simulink model "simulink_model"  (R2019a)
settings: Solver=VariableStepAuto  StartTime=0.0  StopTime=30  RelTol=1e-3
values from neighbouring files (symbols this model uses):
  Kd = 0.28409    [step_10_and_onward.m]
  Ki = 0.05    [step_10_and_onward.m]
  Kp = 1    [P_design.m]    (also in step_10_and_onward.m = 3.12954)
libraries: simulink x1
settings Model: Creator=zma70  LastModifiedBy=zma70

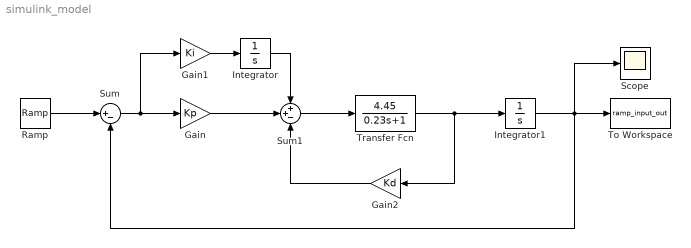
== system simulink_model ==
  Gain : Gain  Gain=Kp
  Gain1 : Gain  Gain=Ki
  Gain2 : Gain  Gain=Kd
  Integrator : Integrator
  Integrator1 : Integrator
  Ramp : simulink/Sources/Ramp  slope=1  start=0  InitialOutput=0
  Scope : Scope
  Sum : Sum  Inputs=|+-
  Sum1 : Sum  Inputs=++-
  To Workspace : ToWorkspace  VariableName=ramp_input_out  SampleTime=-1
      settings: Save2DSignal=2-D array (concatenate along first dimension)
  Transfer Fcn : TransferFcn  Numerator=[4.45]  Denominator=[0.23 1]
  wires:
  Ramp/1 -> Sum/1
  Sum/1 -> Gain1/1, Gain/1
  Gain/1 -> Sum1/2
  Sum1/1 -> Transfer Fcn/1
  Gain1/1 -> Integrator/1
  Integrator/1 -> Sum1/1
  Transfer Fcn/1 -> Gain2/1, Integrator1/1
  Gain2/1 -> Sum1/3
  Integrator1/1 -> Scope/1, Sum/2, To Workspace/1
